simulink subsystem "lift_gas_required_equilibrium"  (R2020a)
settings: Solver=VariableStepAuto  StartTime=0.0  StopTime=10.0  RelTol=1e-3
values from neighbouring files (symbols this model uses):
  M = molar_mass(gas_species)    [calculate_required_gas.m]    (also in configure_simulation.m = molar_mass(lift_gas); evaluate_accel.m; evaluate_jacobian.m; gas_for_equilibrium.m)
  Mair = molar_mass('air')    [configure_simulation.m]
settings Model: Creator=Philip  LastModifiedBy=Philip

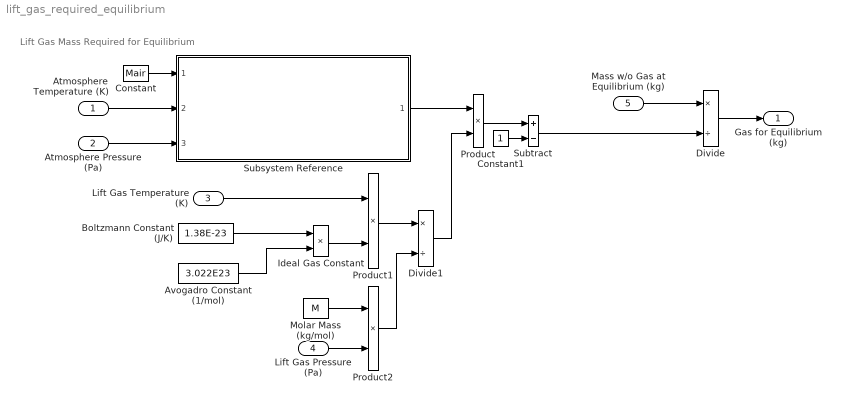
== system lift_gas_required_equilibrium ==
  note: Lift Gas Mass Required for Equilibrium
  Atmosphere Temperature (K) : Inport
  Atmosphere Pressure (Pa) : Inport  Port=2
  Lift Gas Temperature (K) : Inport  Port=3
  Lift Gas Pressure (Pa) : Inport  Port=4
  Mass w/o Gas at Equilibrium (kg) : Inport  Port=5
  Avogadro Constant (1/mol) : Constant  Value=3.022E23
  Boltzmann Constant (J/K) : Constant  Value=1.38E-23
  Constant : Constant  Value=Mair
  Constant1 : Constant
  Divide : Product  Inputs=*/
  Divide1 : Product  Inputs=*/
  Ideal Gas Constant : Product
  Molar Mass (kg/mol) : Constant  Value=M
  Product : Product
  Product1 : Product
  Product2 : Product
  Subsystem Reference : Subsystem  ReferencedSubsystem=rho_ideal
  Subtract : Sum  Inputs=+-
  Gas for Equilibrium (kg) : Outport
  wires:
  Lift Gas Pressure (Pa)/1 -> Product2/2
  Lift Gas Temperature (K)/1 -> Product1/1
  Divide/1 -> Gas for Equilibrium (kg)/1
  Avogadro Constant (1/mol)/1 -> Ideal Gas Constant/2
  Product2/1 -> Divide1/2
  Ideal Gas Constant/1 -> Product1/2
  Boltzmann Constant (J/K)/1 -> Ideal Gas Constant/1
  Molar Mass (kg/mol)/1 -> Product2/1
  Divide1/1 -> Product/2
  Mass w/o Gas at Equilibrium (kg)/1 -> Divide/1
  Product1/1 -> Divide1/1
  Constant/1 -> Subsystem Reference/1
  Atmosphere Temperature (K)/1 -> Subsystem Reference/2
  Atmosphere Pressure (Pa)/1 -> Subsystem Reference/3
  Subsystem Reference/1 -> Product/1
  Product/1 -> Subtract/1
  Constant1/1 -> Subtract/2
  Subtract/1 -> Divide/2
